simulink model "poncy_fuzzy"  (R2025b)
settings: Solver=VariableStepAuto  StartTime=0.0  StopTime=30  RelTol=1e-3
undefined symbols (not defined in the file or in its folder): DiscIntNeverNeededParam
libraries: fuzblock x6, slpidlib x2, simulink x1, sim3dlib x1, uavsim3dlib x1, uavutilslib x1
settings Model: Creator=rel  LastModifiedBy=labro

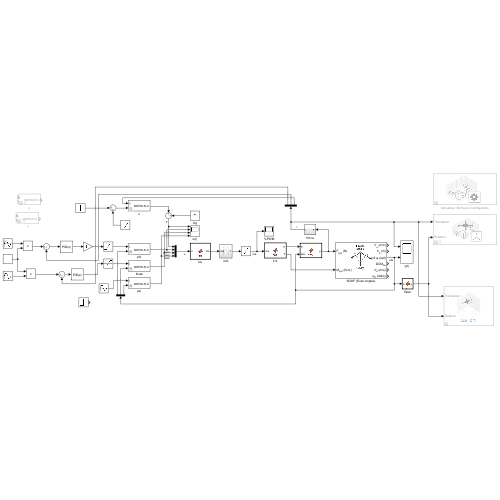
[thumbnail: Simulink's stored preview of the top-level diagram]
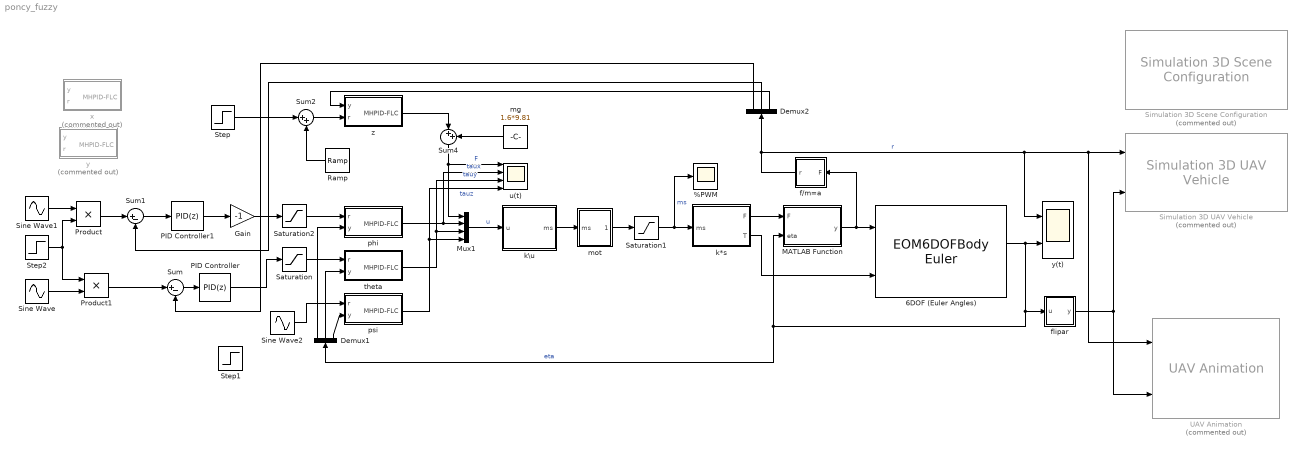
== system poncy_fuzzy ==
  %PWM : Scope
      settings: ActiveDisplayYMinimum=-0.12499999999999997  ActiveDisplayYMaximum=1.125  DataLoggingVariableName=ScopeData4
  6DOF (Euler Angles) : EOM6DOFBodyEuler  mass_0=1.6  inertia=diag([0.021915027 0.022124548 0.042349865])
  Demux1 : Demux  Outputs=3
  Demux2 : Demux  Outputs=3
  Gain : Gain  Gain=-1
  MATLAB Function : MATLAB Function  TreatAsAtomicUnit=on
  Mux1 : Mux
  PID Controller : slpidlib/PID Controller  Controller=PID  Form=Parallel  TimeDomain=Discrete-time  UseExternalTs=off  SampleTime=1/100  IntegratorMethod=Forward Euler  FilterMethod=Forward Euler  ControllerParametersSource=internal  P=0.52  I=0.01  UseKiTs=off  D=0.42  UseExternalDerivativeSource=off  N=100  UseFilter=off  TunerSelectOption=Transfer Function Based (PID Tuner App)  InitialConditionSource=internal  InitialConditionForIntegrator=0  InitialConditionForFilter=0  DifferentiatorICPrevScaledInput=0  ExternalReset=none  TrackingMode=off  Kt=1  LimitOutput=off  SatLimitsSource=internal  UpperSaturationLimit=inf  LowerSaturationLimit=-inf  LinearizeAsGain=on  AntiWindupMode=none  Kb=1  LimitIntegrator=off  UpperIntegratorSaturationLimit=inf  LowerIntegratorSaturationLimit=-inf  POutMin=[]  POutMax=[]  IOutMin=[]  IOutMax=[]  DOutMin=[]  DOutMax=[]  NOutMin=[]  NOutMax=[]  SumOutMin=[]  SumOutMax=[]  SaturationOutMin=[]  SaturationOutMax=[]  PParamMin=[]  PParamMax=[]  IParamMin=[]  IParamMax=[]  DParamMin=[]  DParamMax=[]  NParamMin=[]  NParamMax=[]  KbParamMin=[]  KbParamMax=[]  KtParamMin=[]  KtParamMax=[]  KbOutMin=[]  KbOutMax=[]  KtOutMin=[]  KtOutMax=[]  IntegratorOutMin=[]  IntegratorOutMax=[]  FilterOutMin=[]  FilterOutMax=[]  SumI1OutMin=[]  SumI1OutMax=[]  SumI2OutMin=[]  SumI2OutMax=[]  SumI3OutMin=[]  SumI3OutMax=[]  SumI4OutMin=[]  SumI4OutMax=[]  SumDOutMin=[]  SumDOutMax=[]  DifferentiatorOutMin=[]  DifferentiatorOutMax=[]  FilterDiffOutCoefMin=[]  FilterDiffOutCoefMax=[]  ReciprocalOutMin=[]  ReciprocalOutMax=[]  SumDenOutMin=[]  SumDenOutMax=[]  SumNumOutMin=[]  SumNumOutMax=[]  DivideOutMin=[]  DivideOutMax=[]  UdiffTsProdOutMin=[]  UdiffTsProdOutMax=[]  NTsProdOutMin=[]  NTsProdOutMax=[]  UintegralTsProdOutMin=[]  UintegralTsProdOutMax=[]  UngainTsProdOutMin=[]  UngainTsProdOutMax=[]  ClampingZeroOutDataTypeStr=Inherit: Inherit via back propagation  ClampingZeroOutMin=[]  ClampingZeroOutMax=[]  FilterDenConstantOutDataTypeStr=Inherit: Inherit via back propagation  FilterDenConstantOutMin=[]  FilterDenConstantOutMax=[]  PCopyOutDataTypeStr=Inherit: Inherit via back propagation  PCopyOutMin=[]  PCopyOutMax=[]  NCopyOutDataTypeStr=Inherit: Inherit via back propagation  NCopyOutMin=[]  NCopyOutMax=[]  IntegratorContinuousStateAttributes=''  IntegratorStateMustResolveToSignalObject=off  IntegratorRTWStateStorageClass=Auto  FilterContinuousStateAttributes=''  FilterStateMustResolveToSignalObject=off  FilterRTWStateStorageClass=Auto  ParallelPVariant=InternalParameters  IdealPVariant=Disabled  IVariant=InternalParameters  DVariant=InternalParameters  IntegratorVariant=Discrete  SatVariant=Disabled  AWVariant=Passthrough  PCopyVariant=Disabled  TRVariant=Disabled  FdbkBlocksVariant=Forward  IdealPFdbkVariant=Disabled  SatFdbkVariant=Disabled  DerivativeFilterVariant=Differentiator  NVariant=Passthrough  NCopyVariant=Disabled_SignalSpec  FilterICVariant=InternalICsDifferentiator  IntegratorICVariant=InternalICs  ExternalResetVariant=Disabled  TRSumVariant=Passthrough  SumFdbkVariant=Disabled  SumVariant=Sum_PID  TsampFilterVariant=InternalTs  TsampNgainVariant=Passthrough  TsampIntegralVariant=Disabled_SignalSpec  ExternalSaturationOutDataTypeStr=Inherit: Same as second input  DerivativeSourceVariant=ErrorSignal  PreIntVariant=InternalPreInt
  PID Controller1 : slpidlib/PID Controller  Controller=PID  Form=Parallel  TimeDomain=Discrete-time  UseExternalTs=off  SampleTime=1/100  IntegratorMethod=Forward Euler  FilterMethod=Forward Euler  ControllerParametersSource=internal  P=0.52  I=0.01  UseKiTs=off  D=0.42  UseExternalDerivativeSource=off  N=100  UseFilter=off  TunerSelectOption=Transfer Function Based (PID Tuner App)  InitialConditionSource=internal  InitialConditionForIntegrator=0  InitialConditionForFilter=0  DifferentiatorICPrevScaledInput=0  ExternalReset=none  TrackingMode=off  Kt=1  LimitOutput=off  SatLimitsSource=internal  UpperSaturationLimit=inf  LowerSaturationLimit=-inf  LinearizeAsGain=on  AntiWindupMode=none  Kb=1  LimitIntegrator=off  UpperIntegratorSaturationLimit=inf  LowerIntegratorSaturationLimit=-inf  POutMin=[]  POutMax=[]  IOutMin=[]  IOutMax=[]  DOutMin=[]  DOutMax=[]  NOutMin=[]  NOutMax=[]  SumOutMin=[]  SumOutMax=[]  SaturationOutMin=[]  SaturationOutMax=[]  PParamMin=[]  PParamMax=[]  IParamMin=[]  IParamMax=[]  DParamMin=[]  DParamMax=[]  NParamMin=[]  NParamMax=[]  KbParamMin=[]  KbParamMax=[]  KtParamMin=[]  KtParamMax=[]  KbOutMin=[]  KbOutMax=[]  KtOutMin=[]  KtOutMax=[]  IntegratorOutMin=[]  IntegratorOutMax=[]  FilterOutMin=[]  FilterOutMax=[]  SumI1OutMin=[]  SumI1OutMax=[]  SumI2OutMin=[]  SumI2OutMax=[]  SumI3OutMin=[]  SumI3OutMax=[]  SumI4OutMin=[]  SumI4OutMax=[]  SumDOutMin=[]  SumDOutMax=[]  DifferentiatorOutMin=[]  DifferentiatorOutMax=[]  FilterDiffOutCoefMin=[]  FilterDiffOutCoefMax=[]  ReciprocalOutMin=[]  ReciprocalOutMax=[]  SumDenOutMin=[]  SumDenOutMax=[]  SumNumOutMin=[]  SumNumOutMax=[]  DivideOutMin=[]  DivideOutMax=[]  UdiffTsProdOutMin=[]  UdiffTsProdOutMax=[]  NTsProdOutMin=[]  NTsProdOutMax=[]  UintegralTsProdOutMin=[]  UintegralTsProdOutMax=[]  UngainTsProdOutMin=[]  UngainTsProdOutMax=[]  ClampingZeroOutDataTypeStr=Inherit: Inherit via back propagation  ClampingZeroOutMin=[]  ClampingZeroOutMax=[]  FilterDenConstantOutDataTypeStr=Inherit: Inherit via back propagation  FilterDenConstantOutMin=[]  FilterDenConstantOutMax=[]  PCopyOutDataTypeStr=Inherit: Inherit via back propagation  PCopyOutMin=[]  PCopyOutMax=[]  NCopyOutDataTypeStr=Inherit: Inherit via back propagation  NCopyOutMin=[]  NCopyOutMax=[]  IntegratorContinuousStateAttributes=''  IntegratorStateMustResolveToSignalObject=off  IntegratorRTWStateStorageClass=Auto  FilterContinuousStateAttributes=''  FilterStateMustResolveToSignalObject=off  FilterRTWStateStorageClass=Auto  ParallelPVariant=InternalParameters  IdealPVariant=Disabled  IVariant=InternalParameters  DVariant=InternalParameters  IntegratorVariant=Discrete  SatVariant=Disabled  AWVariant=Passthrough  PCopyVariant=Disabled  TRVariant=Disabled  FdbkBlocksVariant=Forward  IdealPFdbkVariant=Disabled  SatFdbkVariant=Disabled  DerivativeFilterVariant=Differentiator  NVariant=Passthrough  NCopyVariant=Disabled_SignalSpec  FilterICVariant=InternalICsDifferentiator  IntegratorICVariant=InternalICs  ExternalResetVariant=Disabled  TRSumVariant=Passthrough  SumFdbkVariant=Disabled  SumVariant=Sum_PID  TsampFilterVariant=InternalTs  TsampNgainVariant=Passthrough  TsampIntegralVariant=Disabled_SignalSpec  ExternalSaturationOutDataTypeStr=Inherit: Same as second input  DerivativeSourceVariant=ErrorSignal  PreIntVariant=InternalPreInt
  Product : Product
  Product1 : Product
  Ramp : simulink/Sources/Ramp  slope=1/60  start=2  InitialOutput=0
  Saturation : Saturate  UpperLimit=0.9  LowerLimit=-0.9
  Saturation1 : Saturate  UpperLimit=1  LowerLimit=0
  Saturation2 : Saturate  UpperLimit=0.9  LowerLimit=-0.9
  Simulation 3D Scene Configuration : sim3dlib/Simulation 3D Scene Configuration  Priority=0  Commented=on  ProjectFormat=Default Scenes  SceneDesc=US city block  ProjectName=C:\Program Files\MATLAB\R2025b\toolbox\shared\sim3d_projects\automotive_project_windows\UE\WindowsNoEditor\VehicleSimulation.exe  ScenePath=/Game/Maps/USCityBlock  EnableOpenDRIVE=off  vehTagList={'Custom';'Scene Origin';'SimulinkVehicle1'}  vehTag=SimulinkVehicle1  AttachedCameraRelativeTranslation=[0 0 0]  FreeCameraDefaultInitialTranslation=[-6, 0, 2]  AttachedCameraRelativeRotation=[0 0 0]  FreeCameraDefaultInitialRotation=[0, -15, 0]  ViewpointName=Custom  FreeCameraInitialTranslation=[0, 0, 0]  ViewpointTranslation=[0, 0, 0]  FreeCameraInitialRotation=[0, 0, 0]  ViewpointRotation=[0, 0, 0]  OpVisEn=off  Ts=1/60  EnableWindow=on  EnableRemoteAccess=off  EnableWeather=off  SunAzimuth=90  SunAltitude=40.0  EnableGeospatialSun=off  Latitude=0  Longitude=0  Date=2023-01-01  Time=10:30:00  GeoTimeZone=-5.0  SunDaylightSaving=off  wind=1  clouds=10  EnableVolumetricClouds=off  CloudCoverage=0  CloudAltitude=6  fog=0  rain=0  RaindropsEffect=off  SnowDensity=0  EnableGeospatial=off  TilesetSource=Earth terrain  UseTrueOrigin=off  OriginHeight=200  OriginLatitude=40.744652  OriginLongitude=-73.988864  MapStyle=Aerial  AdditionalAssetIDs=[]  UseAdvancedSunSky=off  SolarTime=11  TimeZone=-5  Day=21  Month=9  Year=2022  UseDaylightSavingTime=on  DSTStartDay=10  DSTStartMonth=3  DSTEndDay=3  DSTEndMonth=11  DSTSwitchHour=2  sensorTag=MainCamera1  sensorId=1  sensorName=MainCamera1  mountLoc=Origin  offsetFlag=off  tmountOffset=[0, 0, 0]  rmountOffset=[0, 0, 0]  HorizontalResolution=1280  VerticalResolution=720  HorizontalFOV=60  mountPoint=[0 0 0]  mountOrientation=[0 0 0]  aMode=4  ID=1  GeoTrigger=Inactive  ViewNameList={'Custom'}  ViewTranslationList={'[0 0 0]'}  ViewRotationList={'[0 0 0]'}
      settings: LibrarySourceBlock=uavsim3dlib/Simulation 3D Scene Configuration
  Simulation 3D UAV Vehicle : uavsim3dlib/Simulation 3D UAV Vehicle  Priority=-1  Commented=on  Mesh=Quadrotor  MeshPath=/MathWorksUAVContent/UAVs/HexaRotorUAV/HexaRotor.HexaRotor  Color=Black  ActorName=SimulinkVehicle1  UseGlobalFrame=off  InitialTranslation=[0 0 0]  InitialRotation=[0 0 0]  InitialTranslationGlobal=[0 0 0]  InitialGeoOrigin=[0 0 0]  InitialRotationGlobal=[0 0 0]  SampleTime=-1  ActorType=SimulinkVehicle  ID=1  aMode=4  ActorTag=SimulinkVehicle1
  Sine Wave : Sin  Amplitude=0.5  Bias=0.2  Frequency=3  SampleTime=0
  Sine Wave1 : Sin  Amplitude=0.5  Bias=0.2  Phase=pi/2  SampleTime=0
  Sine Wave2 : Sin  Amplitude=deg2rad(10)  SampleTime=0
  Step : Step  SampleTime=0
  Step1 : Step  Time=3  After=0.5  SampleTime=0
  Step2 : Step  Time=3  After=0.5  SampleTime=0
  Sum : Sum  Inputs=|+-
  Sum1 : Sum  Inputs=|+-
  Sum2 : Sum  Inputs=|++
  Sum4 : Sum  Inputs=|++
  UAV Animation : uavutilslib/UAV Animation  Commented=on  NumUAV=1  DynamicUAVConfig=off  UAVType=Multirotor  UAVSize=1  UAVColor=[1 0 0]  UAVTrajectoryAlpha=1  InertialZDirection=Up  RotationFormat=Euler ZYX  DrawMarkers=off  SampleTime=1/100
  f/m=a : Subsystem
  flipar : MATLAB Function  TreatAsAtomicUnit=on
  k*s : MATLAB Function  TreatAsAtomicUnit=on
  k\u : MATLAB Function  TreatAsAtomicUnit=on
  mg : Constant  Value=1.6*9.81
  mot : Subsystem
  phi : Subsystem  mask{GE=1, GCE=0.25*1.15, GCU=1.2*1.671/1.15, GU=0.3*1.671, c=0}
      mask DialogControl DescGroupVar Prompt: MHPID-FLC
  psi : Subsystem  mask{GE=1, GCE=0.25*1.2, GCU=1.2*3.004/1.2, GU=0.3*3.004, c=0}
      mask DialogControl DescGroupVar Prompt: MHPID-FLC
  theta : Subsystem  mask{GE=1, GCE=0.25*1.15, GCU=1.2*1.687/1.15, GU=0.3*1.687, c=100}
      mask DialogControl DescGroupVar Prompt: MHPID-FLC
  u(t) : Scope  NumInputPorts=4
      settings: ActiveDisplayYMinimum=-20.104353001310926  ActiveDisplayYMaximum=123.50602195698615
  x : Subsystem  Commented=on  mask{GE=1, GCE=0.25*2.77, GCU=1.2*0.6505/2.77, GU=0.3*0.6505, c=0}
      mask DialogControl DescGroupVar Prompt: MHPID-FLC
  y : Subsystem  Commented=on  mask{GE=1, GCE=0.25*1.451, GCU=1.2*2.097/1.451, GU=0.3*2.097, c=0}
      mask DialogControl DescGroupVar Prompt: MHPID-FLC
  y(t) : Scope  NumInputPorts=2
      settings: ActiveDisplayYMinimum=-0.79058058973287282  ActiveDisplayYMaximum=1.7100709049101024
  z : Subsystem  mask{GE=1, GCE=0.25*1.61, GCU=1.2*212.4/1.61, GU=0.3*212.4, c=0}
      mask DialogControl DescGroupVar Prompt: MHPID-FLC
  wires:
  mot/1(Out1) -> Saturation1/1
  k\u/1(ms) -> mot/1(ms)
  Saturation1/1 -> %PWM/1, k*s/1(ms)  "ms"
  MATLAB Function/1(y) -> f/m=a/1(F), 6DOF (Euler Angles)/1
  Mux1/1 -> k\u/1(u)  "u"
  Demux1/1 -> phi/2(y)
  phi/1(MHPID-FLC) -> u(t)/2, Mux1/2  "taux"
  Demux1/2 -> theta/2(y)
  theta/1(MHPID-FLC) -> u(t)/3, Mux1/3  "tauy"
  Demux1/3 -> psi/2(y)
  psi/1(MHPID-FLC) -> u(t)/4, Mux1/4  "tauz"
  Sum4/1 -> u(t)/1, Mux1/1  "F"
  Demux2/3 -> z/1(y)
  6DOF (Euler Angles)/3 -> Demux1/1, MATLAB Function/2(eta), flipar/1(u), y(t)/2  "eta"
  f/m=a/1(r) -> Demux2/1, y(t)/1, UAV Animation/1, Simulation 3D UAV Vehicle/1  "r"
  Demux2/1 -> Sum/2
  Demux2/2 -> Sum1/2
  mg/1 -> Sum4/2
  z/1(MHPID-FLC) -> Sum4/1
  Gain/1 -> Saturation2/1
  Saturation/1 -> theta/1(r)
  PID Controller/1 -> Saturation/1
  k*s/1(F) -> MATLAB Function/1(F)
  k*s/2(T) -> 6DOF (Euler Angles)/2
  Sum/1 -> PID Controller/1
  Saturation2/1 -> phi/1(r)
  Sum1/1 -> PID Controller1/1
  PID Controller1/1 -> Gain/1
  flipar/1(y) -> UAV Animation/2, Simulation 3D UAV Vehicle/2
  Product/1 -> Sum1/1
  Product1/1 -> Sum/1
  Sine Wave/1 -> Product1/2
  Sine Wave1/1 -> Product/1
  Step2/1 -> Product1/1, Product/2
  Sum2/1 -> z/2(r)
  Sine Wave2/1 -> psi/1(r)
  Step/1 -> Sum2/1
  Ramp/1 -> Sum2/2

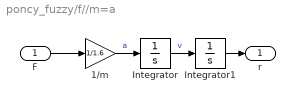
== system poncy_fuzzy/f//m=a ==
  F : Inport
  1/m : Gain  Gain=1/1.6
  Integrator : Integrator
  Integrator1 : Integrator
  r : Outport
  wires:
  Integrator/1 -> Integrator1/1  "v"
  1/m/1 -> Integrator/1  "a"
  F/1 -> 1/m/1
  Integrator1/1 -> r/1

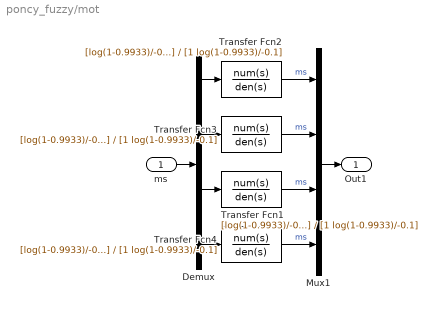
== system poncy_fuzzy/mot ==
  ms : Inport
  Demux : Demux
  Mux1 : Mux
  Transfer Fcn{1..4} (4 alike) : TransferFcn  Numerator=[log(1-0.9933)/-0.1]  Denominator=[1 log(1-0.9933)/-0.1]
  Out1 : Outport
  wires:
  Transfer Fcn3/1 -> Mux1/2  "ms"
  Transfer Fcn1/1 -> Mux1/3  "ms"
  Demux/3 -> Transfer Fcn1/1
  Transfer Fcn4/1 -> Mux1/4  "ms"
  Demux/4 -> Transfer Fcn4/1
  Mux1/1 -> Out1/1
  Transfer Fcn2/1 -> Mux1/1  "ms"
  Demux/2 -> Transfer Fcn3/1
  Demux/1 -> Transfer Fcn2/1
  ms/1 -> Demux/1

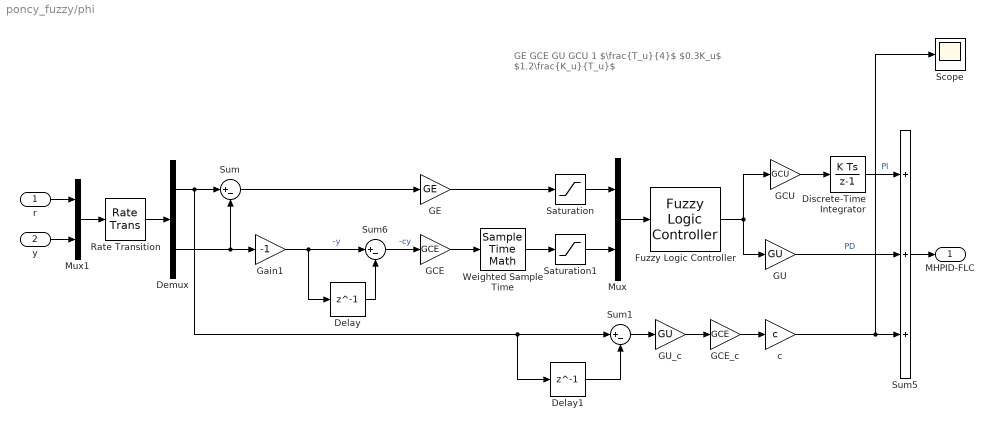
== system poncy_fuzzy/phi ==
  note: GE
      | GCE
      | GU
      | GCU
      |
      | 1
      | $\frac{T_u}{4}$
      | $0.3K_u$
      | $1.2\frac{K_u}{T_u}$
  r : Inport
  y : Inport  Port=2
  Delay : Delay  DelayLength=1
  Delay1 : Delay  DelayLength=1
  Demux : Demux  Outputs=2
  Discrete-Time Integrator : DiscreteIntegrator  SampleTime=-1  ICPrevOutput=DiscIntNeverNeededParam  ICPrevScaledInput=DiscIntNeverNeededParam
  Fuzzy Logic Controller : fuzblock/Fuzzy Logic  Controller  FIS='stfc23.fis'  OutputSampleNumber=101  DataType=double  UseLookupTable=off  NumBreakpoints=10  FuzzifiedInputs=off  RuleFiringStrengths=off  RuleOutputs=off  AggregatedOutputs=off  SimulateUsing=Interpreted execution  OutOfRangeInputValueMessage=warning  NoRuleFiredMessage=warning  EmptyOutputFuzzySetMessage=warning
  GCE : Gain  Gain=GCE
  GCE_c : Gain  Gain=GCE
  GCU : Gain  Gain=GCU
  GE : Gain  Gain=GE
  GU : Gain  Gain=GU
  GU_c : Gain  Gain=GU
  Gain1 : Gain  Gain=-1
  Mux : Mux  Inputs=2
  Mux1 : Mux  Inputs=2
  Rate Transition : RateTransition  OutPortSampleTime=1/100
  Saturation : Saturate  UpperLimit=1  LowerLimit=-1
  Saturation1 : Saturate  UpperLimit=1  LowerLimit=-1
  Scope : Scope
      settings: ActiveDisplayYMinimum=-1  ActiveDisplayYMaximum=1  DataLoggingVariableName=ScopeData2
  Sum : Sum  Inputs=|+-
  Sum1 : Sum  Inputs=|+-
  Sum5 : Sum  Inputs=3
  Sum6 : Sum  Inputs=|+-
  Weighted Sample Time : SampleTimeMath  TsampMathOp=/  weightValue=1
  c : Gain  Gain=c
  MHPID-FLC : Outport
  wires:
  Weighted Sample Time/1 -> Saturation1/1
  Sum6/1 -> GCE/1  "-cy"
  Mux/1 -> Fuzzy Logic Controller/1
  Sum5/1 -> MHPID-FLC/1
  Fuzzy Logic Controller/1 -> GCU/1, GU/1
  Discrete-Time Integrator/1 -> Sum5/1  "PI"
  Delay/1 -> Sum6/2
  Gain1/1 -> Delay/1, Sum6/1  "-y"
  GE/1 -> Saturation/1
  GCE/1 -> Weighted Sample Time/1
  GCU/1 -> Discrete-Time Integrator/1
  GU/1 -> Sum5/2  "PD"
  Sum/1 -> GE/1
  r/1 -> Mux1/1
  y/1 -> Mux1/2
  Mux1/1 -> Rate Transition/1
  Rate Transition/1 -> Demux/1
  Demux/1 -> Delay1/1, Sum1/1, Sum/1
  Demux/2 -> Sum/2, Gain1/1
  Saturation/1 -> Mux/1
  Saturation1/1 -> Mux/2
  GCE_c/1 -> c/1
  GU_c/1 -> GCE_c/1
  Sum1/1 -> GU_c/1
  Delay1/1 -> Sum1/2
  c/1 -> Scope/1, Sum5/3

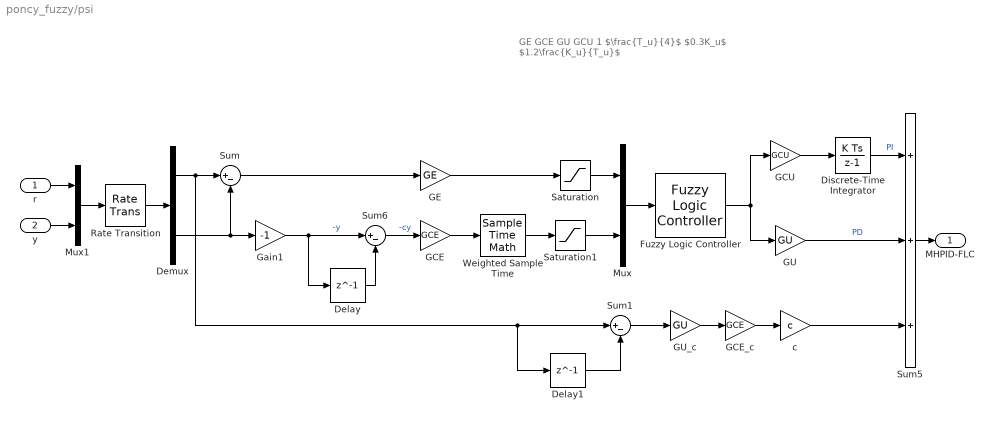
== system poncy_fuzzy/psi ==
  note: GE
      | GCE
      | GU
      | GCU
      |
      | 1
      | $\frac{T_u}{4}$
      | $0.3K_u$
      | $1.2\frac{K_u}{T_u}$
  r : Inport
  y : Inport  Port=2
  Delay : Delay  DelayLength=1
  Delay1 : Delay  DelayLength=1
  Demux : Demux  Outputs=2
  Discrete-Time Integrator : DiscreteIntegrator  SampleTime=-1  ICPrevOutput=DiscIntNeverNeededParam  ICPrevScaledInput=DiscIntNeverNeededParam
  Fuzzy Logic Controller : fuzblock/Fuzzy Logic  Controller  FIS='stfc23.fis'  OutputSampleNumber=101  DataType=double  UseLookupTable=off  NumBreakpoints=10  FuzzifiedInputs=off  RuleFiringStrengths=off  RuleOutputs=off  AggregatedOutputs=off  SimulateUsing=Interpreted execution  OutOfRangeInputValueMessage=warning  NoRuleFiredMessage=warning  EmptyOutputFuzzySetMessage=warning
  GCE : Gain  Gain=GCE
  GCE_c : Gain  Gain=GCE
  GCU : Gain  Gain=GCU
  GE : Gain  Gain=GE
  GU : Gain  Gain=GU
  GU_c : Gain  Gain=GU
  Gain1 : Gain  Gain=-1
  Mux : Mux  Inputs=2
  Mux1 : Mux  Inputs=2
  Rate Transition : RateTransition  OutPortSampleTime=1/100
  Saturation : Saturate  UpperLimit=1  LowerLimit=-1
  Saturation1 : Saturate  UpperLimit=1  LowerLimit=-1
  Sum : Sum  Inputs=|+-
  Sum1 : Sum  Inputs=|+-
  Sum5 : Sum  Inputs=3
  Sum6 : Sum  Inputs=|+-
  Weighted Sample Time : SampleTimeMath  TsampMathOp=/  weightValue=1
  c : Gain  Gain=c
  MHPID-FLC : Outport
  wires:
  Weighted Sample Time/1 -> Saturation1/1
  Sum6/1 -> GCE/1  "-cy"
  Mux/1 -> Fuzzy Logic Controller/1
  Sum5/1 -> MHPID-FLC/1
  Fuzzy Logic Controller/1 -> GCU/1, GU/1
  Discrete-Time Integrator/1 -> Sum5/1  "PI"
  Delay/1 -> Sum6/2
  Gain1/1 -> Delay/1, Sum6/1  "-y"
  GE/1 -> Saturation/1
  GCE/1 -> Weighted Sample Time/1
  GCU/1 -> Discrete-Time Integrator/1
  GU/1 -> Sum5/2  "PD"
  Sum/1 -> GE/1
  r/1 -> Mux1/1
  y/1 -> Mux1/2
  Mux1/1 -> Rate Transition/1
  Rate Transition/1 -> Demux/1
  Demux/2 -> Sum/2, Gain1/1
  Saturation/1 -> Mux/1
  Saturation1/1 -> Mux/2
  GCE_c/1 -> c/1
  Delay1/1 -> Sum1/2
  Sum1/1 -> GU_c/1
  GU_c/1 -> GCE_c/1
  c/1 -> Sum5/3
  Demux/1 -> Delay1/1, Sum1/1, Sum/1

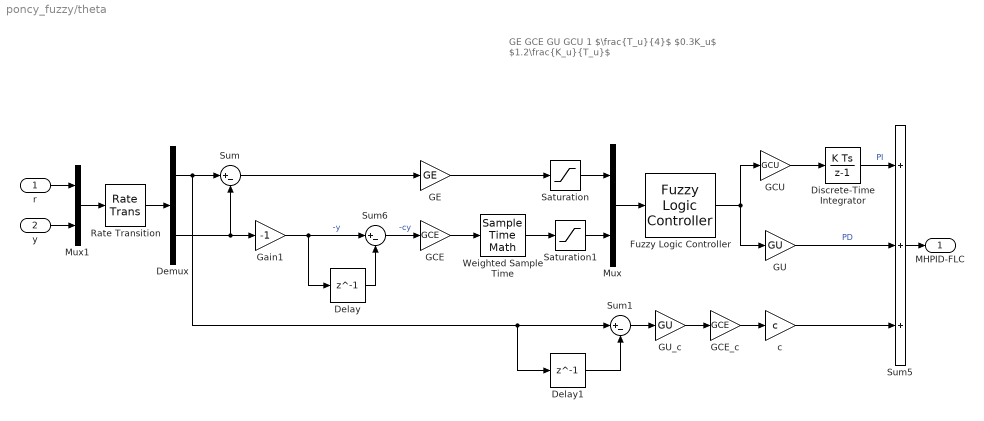
== system poncy_fuzzy/theta ==
  note: GE
      | GCE
      | GU
      | GCU
      |
      | 1
      | $\frac{T_u}{4}$
      | $0.3K_u$
      | $1.2\frac{K_u}{T_u}$
  r : Inport
  y : Inport  Port=2
  Delay : Delay  DelayLength=1
  Delay1 : Delay  DelayLength=1
  Demux : Demux  Outputs=2
  Discrete-Time Integrator : DiscreteIntegrator  SampleTime=-1  ICPrevOutput=DiscIntNeverNeededParam  ICPrevScaledInput=DiscIntNeverNeededParam
  Fuzzy Logic Controller : fuzblock/Fuzzy Logic  Controller  FIS='stfc23.fis'  OutputSampleNumber=101  DataType=double  UseLookupTable=off  NumBreakpoints=10  FuzzifiedInputs=off  RuleFiringStrengths=off  RuleOutputs=off  AggregatedOutputs=off  SimulateUsing=Interpreted execution  OutOfRangeInputValueMessage=warning  NoRuleFiredMessage=warning  EmptyOutputFuzzySetMessage=warning
  GCE : Gain  Gain=GCE
  GCE_c : Gain  Gain=GCE
  GCU : Gain  Gain=GCU
  GE : Gain  Gain=GE
  GU : Gain  Gain=GU
  GU_c : Gain  Gain=GU
  Gain1 : Gain  Gain=-1
  Mux : Mux  Inputs=2
  Mux1 : Mux  Inputs=2
  Rate Transition : RateTransition  OutPortSampleTime=1/100
  Saturation : Saturate  UpperLimit=1  LowerLimit=-1
  Saturation1 : Saturate  UpperLimit=1  LowerLimit=-1
  Sum : Sum  Inputs=|+-
  Sum1 : Sum  Inputs=|+-
  Sum5 : Sum  Inputs=3
  Sum6 : Sum  Inputs=|+-
  Weighted Sample Time : SampleTimeMath  TsampMathOp=/  weightValue=1
  c : Gain  Gain=c
  MHPID-FLC : Outport
  wires:
  Weighted Sample Time/1 -> Saturation1/1
  Sum6/1 -> GCE/1  "-cy"
  Mux/1 -> Fuzzy Logic Controller/1
  Sum5/1 -> MHPID-FLC/1
  Fuzzy Logic Controller/1 -> GCU/1, GU/1
  Discrete-Time Integrator/1 -> Sum5/1  "PI"
  Delay/1 -> Sum6/2
  Gain1/1 -> Delay/1, Sum6/1  "-y"
  GE/1 -> Saturation/1
  GCE/1 -> Weighted Sample Time/1
  GCU/1 -> Discrete-Time Integrator/1
  GU/1 -> Sum5/2  "PD"
  Sum/1 -> GE/1
  r/1 -> Mux1/1
  y/1 -> Mux1/2
  Mux1/1 -> Rate Transition/1
  Rate Transition/1 -> Demux/1
  Demux/2 -> Sum/2, Gain1/1
  Saturation/1 -> Mux/1
  Saturation1/1 -> Mux/2
  GU_c/1 -> GCE_c/1
  c/1 -> Sum5/3
  Delay1/1 -> Sum1/2
  GCE_c/1 -> c/1
  Demux/1 -> Delay1/1, Sum1/1, Sum/1
  Sum1/1 -> GU_c/1

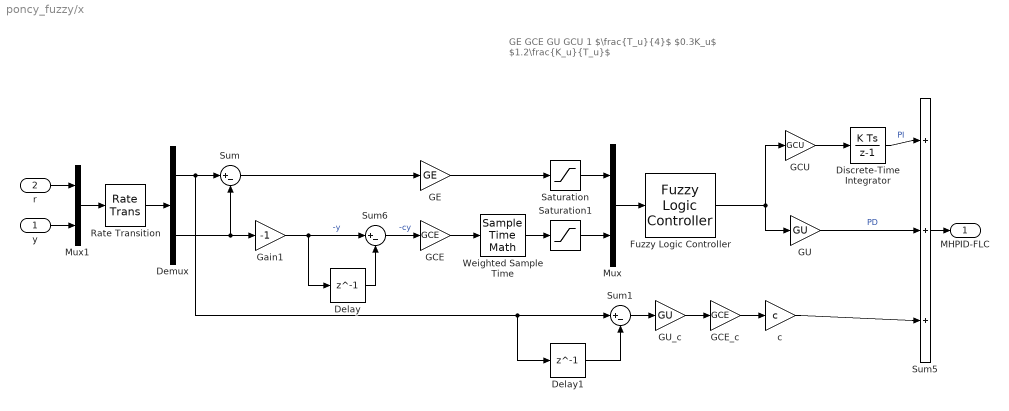
== system poncy_fuzzy/x ==
  note: GE
      | GCE
      | GU
      | GCU
      |
      | 1
      | $\frac{T_u}{4}$
      | $0.3K_u$
      | $1.2\frac{K_u}{T_u}$
  y : Inport
  r : Inport  Port=2
  Delay : Delay  DelayLength=1
  Delay1 : Delay  DelayLength=1
  Demux : Demux  Outputs=2
  Discrete-Time Integrator : DiscreteIntegrator  SampleTime=-1  ICPrevOutput=DiscIntNeverNeededParam  ICPrevScaledInput=DiscIntNeverNeededParam
  Fuzzy Logic Controller : fuzblock/Fuzzy Logic  Controller  FIS='stfc23.fis'  OutputSampleNumber=101  DataType=double  UseLookupTable=off  NumBreakpoints=10  FuzzifiedInputs=off  RuleFiringStrengths=off  RuleOutputs=off  AggregatedOutputs=off  SimulateUsing=Interpreted execution  OutOfRangeInputValueMessage=warning  NoRuleFiredMessage=warning  EmptyOutputFuzzySetMessage=warning
  GCE : Gain  Gain=GCE
  GCE_c : Gain  Gain=GCE
  GCU : Gain  Gain=GCU
  GE : Gain  Gain=GE
  GU : Gain  Gain=GU
  GU_c : Gain  Gain=GU
  Gain1 : Gain  Gain=-1
  Mux : Mux  Inputs=2
  Mux1 : Mux  Inputs=2
  Rate Transition : RateTransition  OutPortSampleTime=1/100
  Saturation : Saturate  UpperLimit=1  LowerLimit=-1
  Saturation1 : Saturate  UpperLimit=1  LowerLimit=-1
  Sum : Sum  Inputs=|+-
  Sum1 : Sum  Inputs=|+-
  Sum5 : Sum  Inputs=3
  Sum6 : Sum  Inputs=|+-
  Weighted Sample Time : SampleTimeMath  TsampMathOp=/  weightValue=1
  c : Gain  Gain=c
  MHPID-FLC : Outport
  wires:
  Weighted Sample Time/1 -> Saturation1/1
  Sum6/1 -> GCE/1  "-cy"
  Mux/1 -> Fuzzy Logic Controller/1
  Sum5/1 -> MHPID-FLC/1
  Fuzzy Logic Controller/1 -> GU/1, GCU/1
  Discrete-Time Integrator/1 -> Sum5/1  "PI"
  Delay/1 -> Sum6/2
  Gain1/1 -> Delay/1, Sum6/1  "-y"
  GE/1 -> Saturation/1
  GCE/1 -> Weighted Sample Time/1
  GCU/1 -> Discrete-Time Integrator/1
  GU/1 -> Sum5/2  "PD"
  Sum/1 -> GE/1
  r/1 -> Mux1/1
  y/1 -> Mux1/2
  Mux1/1 -> Rate Transition/1
  Rate Transition/1 -> Demux/1
  Demux/2 -> Sum/2, Gain1/1
  Saturation/1 -> Mux/1
  Saturation1/1 -> Mux/2
  GCE_c/1 -> c/1
  GU_c/1 -> GCE_c/1
  Sum1/1 -> GU_c/1
  Demux/1 -> Delay1/1, Sum1/1, Sum/1
  Delay1/1 -> Sum1/2
  c/1 -> Sum5/3

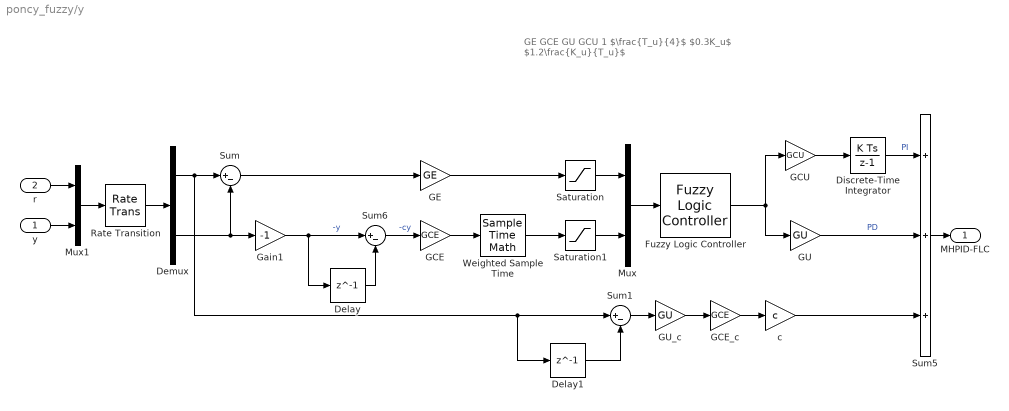
== system poncy_fuzzy/y ==
  note: GE
      | GCE
      | GU
      | GCU
      |
      | 1
      | $\frac{T_u}{4}$
      | $0.3K_u$
      | $1.2\frac{K_u}{T_u}$
  y : Inport
  r : Inport  Port=2
  Delay : Delay  DelayLength=1
  Delay1 : Delay  DelayLength=1
  Demux : Demux  Outputs=2
  Discrete-Time Integrator : DiscreteIntegrator  SampleTime=-1  ICPrevOutput=DiscIntNeverNeededParam  ICPrevScaledInput=DiscIntNeverNeededParam
  Fuzzy Logic Controller : fuzblock/Fuzzy Logic  Controller  FIS='stfc23.fis'  OutputSampleNumber=101  DataType=double  UseLookupTable=off  NumBreakpoints=10  FuzzifiedInputs=off  RuleFiringStrengths=off  RuleOutputs=off  AggregatedOutputs=off  SimulateUsing=Interpreted execution  OutOfRangeInputValueMessage=warning  NoRuleFiredMessage=warning  EmptyOutputFuzzySetMessage=warning
  GCE : Gain  Gain=GCE
  GCE_c : Gain  Gain=GCE
  GCU : Gain  Gain=GCU
  GE : Gain  Gain=GE
  GU : Gain  Gain=GU
  GU_c : Gain  Gain=GU
  Gain1 : Gain  Gain=-1
  Mux : Mux  Inputs=2
  Mux1 : Mux  Inputs=2
  Rate Transition : RateTransition  OutPortSampleTime=1/100
  Saturation : Saturate  UpperLimit=1  LowerLimit=-1
  Saturation1 : Saturate  UpperLimit=1  LowerLimit=-1
  Sum : Sum  Inputs=|+-
  Sum1 : Sum  Inputs=|+-
  Sum5 : Sum  Inputs=3
  Sum6 : Sum  Inputs=|+-
  Weighted Sample Time : SampleTimeMath  TsampMathOp=/  weightValue=1
  c : Gain  Gain=c
  MHPID-FLC : Outport
  wires:
  Weighted Sample Time/1 -> Saturation1/1
  Sum6/1 -> GCE/1  "-cy"
  Mux/1 -> Fuzzy Logic Controller/1
  Sum5/1 -> MHPID-FLC/1
  Fuzzy Logic Controller/1 -> GU/1, GCU/1
  Discrete-Time Integrator/1 -> Sum5/1  "PI"
  Delay/1 -> Sum6/2
  Gain1/1 -> Delay/1, Sum6/1  "-y"
  GE/1 -> Saturation/1
  GCE/1 -> Weighted Sample Time/1
  GCU/1 -> Discrete-Time Integrator/1
  GU/1 -> Sum5/2  "PD"
  Sum/1 -> GE/1
  r/1 -> Mux1/1
  y/1 -> Mux1/2
  Mux1/1 -> Rate Transition/1
  Rate Transition/1 -> Demux/1
  Demux/2 -> Sum/2, Gain1/1
  Saturation/1 -> Mux/1
  Saturation1/1 -> Mux/2
  GCE_c/1 -> c/1
  GU_c/1 -> GCE_c/1
  Sum1/1 -> GU_c/1
  Demux/1 -> Delay1/1, Sum1/1, Sum/1
  Delay1/1 -> Sum1/2
  c/1 -> Sum5/3

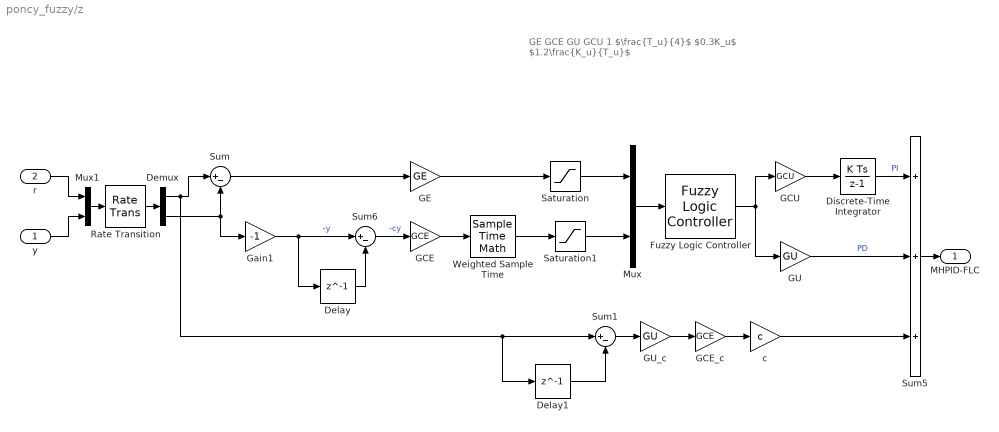
== system poncy_fuzzy/z ==
  note: GE
      | GCE
      | GU
      | GCU
      |
      | 1
      | $\frac{T_u}{4}$
      | $0.3K_u$
      | $1.2\frac{K_u}{T_u}$
  y : Inport
  r : Inport  Port=2
  Delay : Delay  DelayLength=1
  Delay1 : Delay  DelayLength=1
  Demux : Demux  Outputs=2
  Discrete-Time Integrator : DiscreteIntegrator  SampleTime=-1  ICPrevOutput=DiscIntNeverNeededParam  ICPrevScaledInput=DiscIntNeverNeededParam
  Fuzzy Logic Controller : fuzblock/Fuzzy Logic  Controller  FIS='stfc23.fis'  OutputSampleNumber=101  DataType=double  UseLookupTable=off  NumBreakpoints=10  FuzzifiedInputs=off  RuleFiringStrengths=off  RuleOutputs=off  AggregatedOutputs=off  SimulateUsing=Interpreted execution  OutOfRangeInputValueMessage=warning  NoRuleFiredMessage=warning  EmptyOutputFuzzySetMessage=warning
  GCE : Gain  Gain=GCE
  GCE_c : Gain  Gain=GCE
  GCU : Gain  Gain=GCU
  GE : Gain  Gain=GE
  GU : Gain  Gain=GU
  GU_c : Gain  Gain=GU
  Gain1 : Gain  Gain=-1
  Mux : Mux  Inputs=2
  Mux1 : Mux  Inputs=2
  Rate Transition : RateTransition  OutPortSampleTime=1/100
  Saturation : Saturate  UpperLimit=1  LowerLimit=-1
  Saturation1 : Saturate  UpperLimit=1  LowerLimit=-1
  Sum : Sum  Inputs=|+-
  Sum1 : Sum  Inputs=|+-
  Sum5 : Sum  Inputs=3
  Sum6 : Sum  Inputs=|+-
  Weighted Sample Time : SampleTimeMath  TsampMathOp=/  weightValue=1
  c : Gain  Gain=c
  MHPID-FLC : Outport
  wires:
  Weighted Sample Time/1 -> Saturation1/1
  Sum6/1 -> GCE/1  "-cy"
  Mux/1 -> Fuzzy Logic Controller/1
  Sum5/1 -> MHPID-FLC/1
  Fuzzy Logic Controller/1 -> GCU/1, GU/1
  Discrete-Time Integrator/1 -> Sum5/1  "PI"
  Delay/1 -> Sum6/2
  Gain1/1 -> Delay/1, Sum6/1  "-y"
  GE/1 -> Saturation/1
  GCE/1 -> Weighted Sample Time/1
  GCU/1 -> Discrete-Time Integrator/1
  GU/1 -> Sum5/2  "PD"
  Sum/1 -> GE/1
  y/1 -> Mux1/2
  Demux/2 -> Gain1/1, Sum/2
  Mux1/1 -> Rate Transition/1
  r/1 -> Mux1/1
  Rate Transition/1 -> Demux/1
  Saturation/1 -> Mux/1
  Saturation1/1 -> Mux/2
  GU_c/1 -> GCE_c/1
  c/1 -> Sum5/3
  Delay1/1 -> Sum1/2
  Demux/1 -> Delay1/1, Sum1/1, Sum/1
  Sum1/1 -> GU_c/1
  GCE_c/1 -> c/1

== matlab function poncy_fuzzy/k\u ==
  data: u input; ms output
function ms = fcn(u)
% L = 0.0080;
% kF = 0.1600*9.81;
% kM = 0.0086;
L = 0.268554;
kF = 0.7*9.81;
kM = 0.2;
A = [kF kF kF kF;
    -L*kF -L*kF L*kF L*kF;
    -L*kF L*kF L*kF -L*kF;
    -kM kM -kM kM];
ms = A\u;

== matlab function poncy_fuzzy/MATLAB Function ==
  data: F input; y output; eta input
function y = fcn(F, eta)
phi = eta(1);
theta = eta(2);
psi = eta(3);
y = [0;0;-1.6*9.81] + [sin(theta)*cos(psi) + sin(phi)*cos(theta)*sin(psi); ...
                    sin(theta)*sin(psi) - sin(phi)*cos(theta)*cos(psi); ...
                    cos(phi)*cos(theta)]*F;

== matlab function poncy_fuzzy/k*s ==
  data: ms input; F output; T output
function [F, T] = fcn(ms)
% L = 0.0080;
% kF = 0.1600*9.81;
% kM = 0.0086;
L = 0.268554;
kF = 0.7*9.81;
kM = 0.2;
A = [kF kF kF kF;
    -L*kF -L*kF L*kF L*kF;
    -L*kF L*kF L*kF -L*kF;
    -kM kM -kM kM];
y = A*ms;
F = y(1);
T = y(2:end);

== matlab function poncy_fuzzy/flipar ==
  data: u input; y output
function y = fcn(u)
y = flip(u);
